simulink model "TST_InjSys_CtlQnt"  (R2016b)
settings: Solver=FixedStepDiscrete  StartTime=0.0  StopTime=simTime  FixedStep=sampleTime  RelTol=1e-3
values from neighbouring files (symbols this model uses):
  testCase = 1    [initTST_InjSys_CtlQnt_001.m]
libraries: simulink x4, UnitTest_Lib x2
settings Model: Creator=zhengjinyan  LastModifiedBy=zhengjinyan
settings DebuggingCC: SignalRangeChecking=error

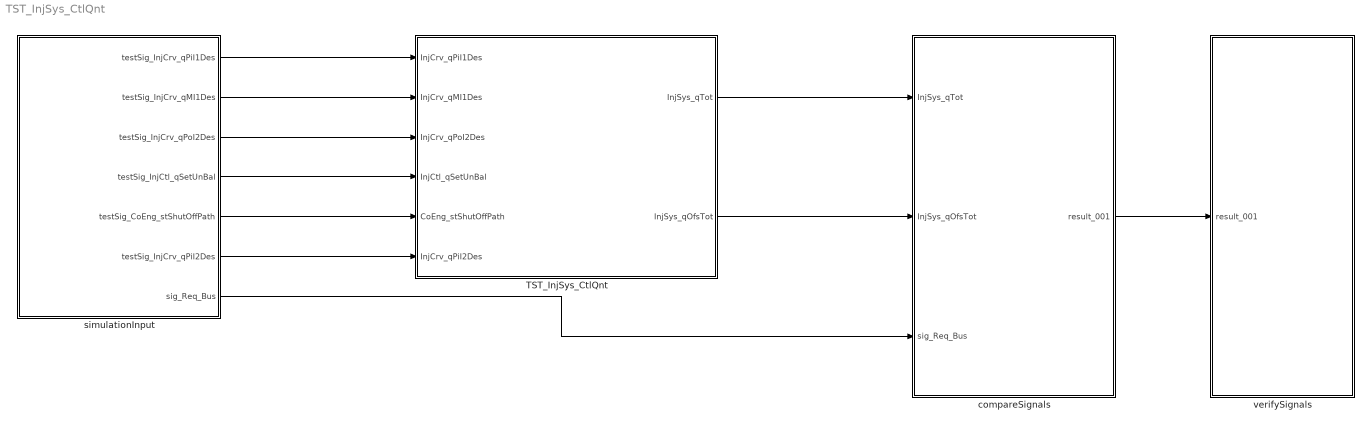
== system TST_InjSys_CtlQnt ==
  TST_InjSys_CtlQnt : Subsystem
  compareSignals : Subsystem
  simulationInput : Subsystem
  verifySignals : Subsystem
  wires:
  simulationInput/1(testSig_InjCrv_qPiI1Des) -> TST_InjSys_CtlQnt/1(InjCrv_qPiI1Des)
  simulationInput/2(testSig_InjCrv_qMI1Des) -> TST_InjSys_CtlQnt/2(InjCrv_qMI1Des)
  simulationInput/3(testSig_InjCrv_qPoI2Des) -> TST_InjSys_CtlQnt/3(InjCrv_qPoI2Des)
  simulationInput/4(testSig_InjCtl_qSetUnBal) -> TST_InjSys_CtlQnt/4(InjCtl_qSetUnBal)
  simulationInput/5(testSig_CoEng_stShutOffPath) -> TST_InjSys_CtlQnt/5(CoEng_stShutOffPath)
  simulationInput/6(testSig_InjCrv_qPiI2Des) -> TST_InjSys_CtlQnt/6(InjCrv_qPiI2Des)
  TST_InjSys_CtlQnt/1(InjSys_qTot) -> compareSignals/1(InjSys_qTot)
  TST_InjSys_CtlQnt/2(InjSys_qOfsTot) -> compareSignals/2(InjSys_qOfsTot)
  simulationInput/7(sig_Req_Bus) -> compareSignals/3(sig_Req_Bus)
  compareSignals/1(result_001) -> verifySignals/1(result_001)

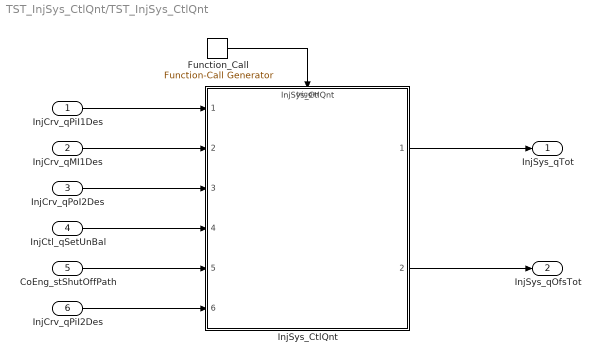
== system TST_InjSys_CtlQnt/TST_InjSys_CtlQnt ==
  InjCrv_qPiI1Des : Inport
  InjCrv_qMI1Des : Inport  Port=2
  InjCrv_qPoI2Des : Inport  Port=3
  InjCtl_qSetUnBal : Inport  Port=4
  CoEng_stShutOffPath : Inport  Port=5
  InjCrv_qPiI2Des : Inport  Port=6
  Function_Call : simulink/Ports & Subsystems/Function-Call Generator  sample_time=sampleTime  numberOfIterations=1
  InjSys_CtlQnt : ModelReference  ModelNameDialog=InjSys_CtlQnt  SimulationMode=Normal  ModelReferenceVersion=1.5  TriggerPortName=function  TriggerPortTriggerType=function-call  TriggerPortStatesWhenEnabling=held
  InjSys_qTot : Outport
  InjSys_qOfsTot : Outport  Port=2
  wires:
  Function_Call/1 -> InjSys_CtlQnt/Trigger
  InjCrv_qPiI1Des/1 -> InjSys_CtlQnt/1
  InjCrv_qMI1Des/1 -> InjSys_CtlQnt/2
  InjCrv_qPoI2Des/1 -> InjSys_CtlQnt/3
  InjCtl_qSetUnBal/1 -> InjSys_CtlQnt/4
  CoEng_stShutOffPath/1 -> InjSys_CtlQnt/5
  InjCrv_qPiI2Des/1 -> InjSys_CtlQnt/6
  InjSys_CtlQnt/1 -> InjSys_qTot/1
  InjSys_CtlQnt/2 -> InjSys_qOfsTot/1

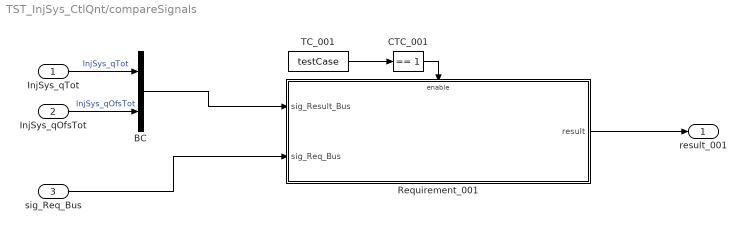
== system TST_InjSys_CtlQnt/compareSignals ==
  InjSys_qTot : Inport
  InjSys_qOfsTot : Inport  Port=2
  sig_Req_Bus : Inport  Port=3
  BC : BusCreator  Inputs=2
  CTC_001 : simulink/Logic and Bit Operations/Compare To Constant  relop===  const=1  OutDataTypeStr=boolean
  Requirement_001 : Subsystem
  TC_001 : Constant  Value=testCase
  result_001 : Outport
  wires:
  InjSys_qTot/1 -> BC/1  "InjSys_qTot"
  InjSys_qOfsTot/1 -> BC/2  "InjSys_qOfsTot"
  TC_001/1 -> CTC_001/1
  CTC_001/1 -> Requirement_001/Enable
  sig_Req_Bus/1 -> Requirement_001/2(sig_Req_Bus)
  BC/1 -> Requirement_001/1(sig_Result_Bus)
  Requirement_001/1(result) -> result_001/1

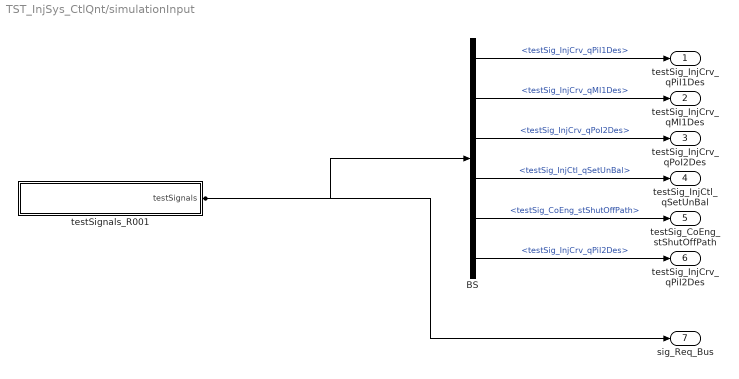
== system TST_InjSys_CtlQnt/simulationInput ==
  BS : BusSelector  OutputSignals=testSig_InjCrv_qPiI1Des,testSig_InjCrv_qMI1Des,testSig_InjCrv_qPoI2Des,testSig_InjCtl_qSetUnBal,testSig_CoEng_stShutOffPath,testSig_InjCrv_qPiI2Des
  testSignals_R001 : Subsystem
  testSig_InjCrv_qPiI1Des : Outport
  testSig_InjCrv_qMI1Des : Outport  Port=2
  testSig_InjCrv_qPoI2Des : Outport  Port=3
  testSig_InjCtl_qSetUnBal : Outport  Port=4
  testSig_CoEng_stShutOffPath : Outport  Port=5
  testSig_InjCrv_qPiI2Des : Outport  Port=6
  sig_Req_Bus : Outport  Port=7
  wires:
  BS/1 -> testSig_InjCrv_qPiI1Des/1  "<testSig_InjCrv_qPiI1Des>"
  BS/2 -> testSig_InjCrv_qMI1Des/1  "<testSig_InjCrv_qMI1Des>"
  BS/3 -> testSig_InjCrv_qPoI2Des/1  "<testSig_InjCrv_qPoI2Des>"
  BS/4 -> testSig_InjCtl_qSetUnBal/1  "<testSig_InjCtl_qSetUnBal>"
  BS/5 -> testSig_CoEng_stShutOffPath/1  "<testSig_CoEng_stShutOffPath>"
  BS/6 -> testSig_InjCrv_qPiI2Des/1  "<testSig_InjCrv_qPiI2Des>"
  testSignals_R001/1(testSignals) -> BS/1, sig_Req_Bus/1

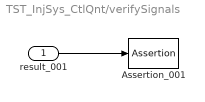
== system TST_InjSys_CtlQnt/verifySignals ==
  result_001 : Inport
  Assertion_001 : Assertion  Enabled=off
  wires:
  result_001/1 -> Assertion_001/1

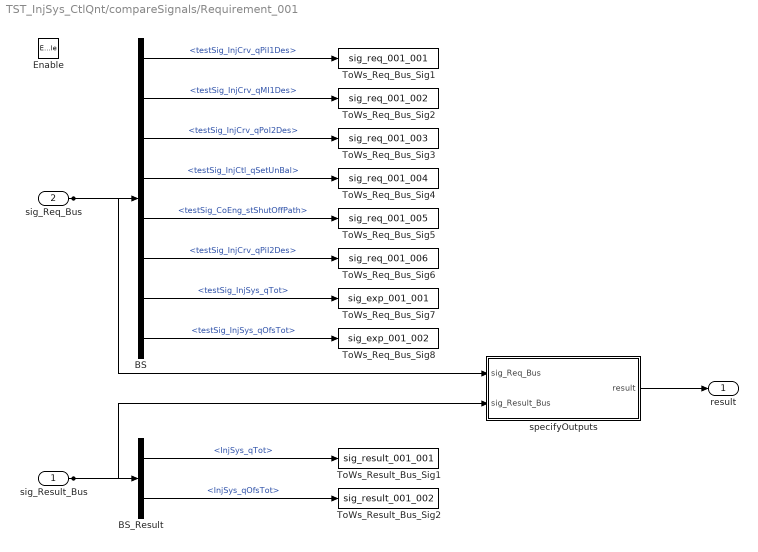
== system TST_InjSys_CtlQnt/compareSignals/Requirement_001 ==
  sig_Result_Bus : Inport
  sig_Req_Bus : Inport  Port=2
  Enable : EnablePort
  BS : BusSelector  OutputSignals=testSig_InjCrv_qPiI1Des,testSig_InjCrv_qMI1Des,testSig_InjCrv_qPoI2Des,testSig_InjCtl_qSetUnBal,testSig_CoEng_stShutOffPath,testSig_InjCrv_qPiI2Des,testSig_InjSys_qTot,testSig_InjSys_qOfsTot
  BS_Result : BusSelector  OutputSignals=InjSys_qTot,InjSys_qOfsTot
  ToWs_Req_Bus_Sig1 : ToWorkspace  VariableName=sig_req_001_001  SaveFormat=Structure With Time
  ToWs_Req_Bus_Sig2 : ToWorkspace  VariableName=sig_req_001_002  SaveFormat=Structure With Time
  ToWs_Req_Bus_Sig3 : ToWorkspace  VariableName=sig_req_001_003  SaveFormat=Structure With Time
  ToWs_Req_Bus_Sig4 : ToWorkspace  VariableName=sig_req_001_004  SaveFormat=Structure With Time
  ToWs_Req_Bus_Sig5 : ToWorkspace  VariableName=sig_req_001_005  SaveFormat=Structure With Time
  ToWs_Req_Bus_Sig6 : ToWorkspace  VariableName=sig_req_001_006  SaveFormat=Structure With Time
  ToWs_Req_Bus_Sig7 : ToWorkspace  VariableName=sig_exp_001_001  SaveFormat=Structure With Time
  ToWs_Req_Bus_Sig8 : ToWorkspace  VariableName=sig_exp_001_002  SaveFormat=Structure With Time
  ToWs_Result_Bus_Sig1 : ToWorkspace  VariableName=sig_result_001_001  SaveFormat=Structure With Time
  ToWs_Result_Bus_Sig2 : ToWorkspace  VariableName=sig_result_001_002  SaveFormat=Structure With Time
  specifyOutputs : Subsystem
  result : Outport
  wires:
  sig_Req_Bus/1 -> BS/1, specifyOutputs/1(sig_Req_Bus)
  BS/1 -> ToWs_Req_Bus_Sig1/1  "<testSig_InjCrv_qPiI1Des>"
  BS/2 -> ToWs_Req_Bus_Sig2/1  "<testSig_InjCrv_qMI1Des>"
  BS/3 -> ToWs_Req_Bus_Sig3/1  "<testSig_InjCrv_qPoI2Des>"
  BS/4 -> ToWs_Req_Bus_Sig4/1  "<testSig_InjCtl_qSetUnBal>"
  BS/5 -> ToWs_Req_Bus_Sig5/1  "<testSig_CoEng_stShutOffPath>"
  BS/6 -> ToWs_Req_Bus_Sig6/1  "<testSig_InjCrv_qPiI2Des>"
  BS/7 -> ToWs_Req_Bus_Sig7/1  "<testSig_InjSys_qTot>"
  BS/8 -> ToWs_Req_Bus_Sig8/1  "<testSig_InjSys_qOfsTot>"
  sig_Result_Bus/1 -> BS_Result/1, specifyOutputs/2(sig_Result_Bus)
  BS_Result/1 -> ToWs_Result_Bus_Sig1/1  "<InjSys_qTot>"
  BS_Result/2 -> ToWs_Result_Bus_Sig2/1  "<InjSys_qOfsTot>"
  specifyOutputs/1(result) -> result/1

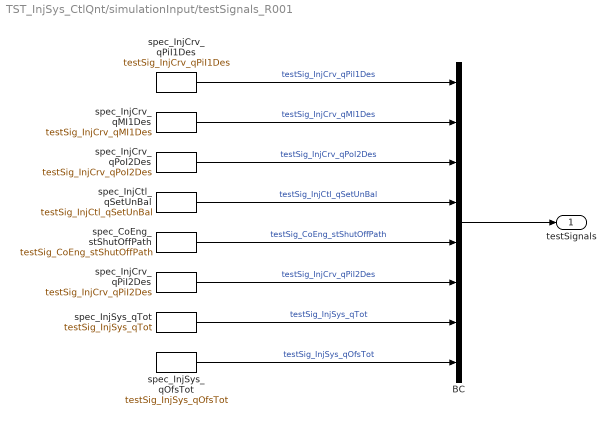
== system TST_InjSys_CtlQnt/simulationInput/testSignals_R001 ==
  BC : BusCreator  Inputs=8
  spec_CoEng_stShutOffPath : FromWorkspace  VariableName=testSig_CoEng_stShutOffPath  Interpolate=off  OutputAfterFinalValue=Holding final value
  spec_InjCrv_qMI1Des : FromWorkspace  VariableName=testSig_InjCrv_qMI1Des  Interpolate=off  OutputAfterFinalValue=Holding final value
  spec_InjCrv_qPiI1Des : FromWorkspace  VariableName=testSig_InjCrv_qPiI1Des  Interpolate=off  OutputAfterFinalValue=Holding final value
  spec_InjCrv_qPiI2Des : FromWorkspace  VariableName=testSig_InjCrv_qPiI2Des  Interpolate=off  OutputAfterFinalValue=Holding final value
  spec_InjCrv_qPoI2Des : FromWorkspace  VariableName=testSig_InjCrv_qPoI2Des  Interpolate=off  OutputAfterFinalValue=Holding final value
  spec_InjCtl_qSetUnBal : FromWorkspace  VariableName=testSig_InjCtl_qSetUnBal  Interpolate=off  OutputAfterFinalValue=Holding final value
  spec_InjSys_qOfsTot : FromWorkspace  VariableName=testSig_InjSys_qOfsTot  Interpolate=off  OutputAfterFinalValue=Holding final value
  spec_InjSys_qTot : FromWorkspace  VariableName=testSig_InjSys_qTot  Interpolate=off  OutputAfterFinalValue=Holding final value
  testSignals : Outport
  wires:
  BC/1 -> testSignals/1
  spec_InjCrv_qPiI1Des/1 -> BC/1  "testSig_InjCrv_qPiI1Des"
  spec_InjCrv_qMI1Des/1 -> BC/2  "testSig_InjCrv_qMI1Des"
  spec_InjCrv_qPoI2Des/1 -> BC/3  "testSig_InjCrv_qPoI2Des"
  spec_InjCtl_qSetUnBal/1 -> BC/4  "testSig_InjCtl_qSetUnBal"
  spec_CoEng_stShutOffPath/1 -> BC/5  "testSig_CoEng_stShutOffPath"
  spec_InjCrv_qPiI2Des/1 -> BC/6  "testSig_InjCrv_qPiI2Des"
  spec_InjSys_qTot/1 -> BC/7  "testSig_InjSys_qTot"
  spec_InjSys_qOfsTot/1 -> BC/8  "testSig_InjSys_qOfsTot"

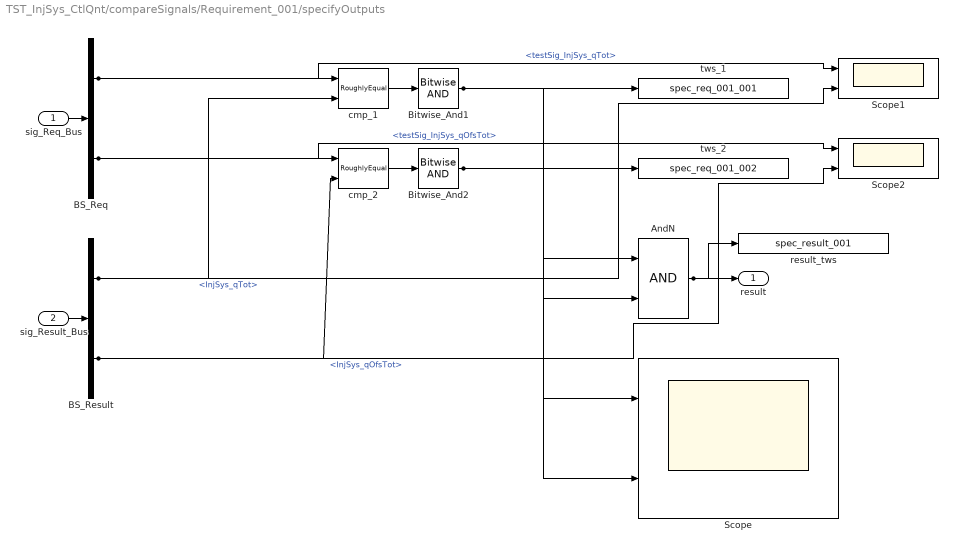
== system TST_InjSys_CtlQnt/compareSignals/Requirement_001/specifyOutputs ==
  sig_Req_Bus : Inport
  sig_Result_Bus : Inport  Port=2
  AndN : Logic
  BS_Req : BusSelector  OutputSignals=testSig_InjSys_qTot,testSig_InjSys_qOfsTot
  BS_Result : BusSelector  OutputSignals=InjSys_qTot,InjSys_qOfsTot
  Bitwise_And1 : simulink/Logic and Bit Operations/Bitwise Operator  logicop=AND  UseBitMask=off  BitMask=bin2dec('11011001')  BitMaskRealWorld=Stored Integer
  Bitwise_And2 : simulink/Logic and Bit Operations/Bitwise Operator  logicop=AND  UseBitMask=off  BitMask=bin2dec('11011001')  BitMaskRealWorld=Stored Integer
  Scope : Scope  NumInputPorts=2
  Scope1 : Scope  NumInputPorts=2
  Scope2 : Scope  NumInputPorts=2
  cmp_1 : UnitTest_Lib/RoughlyEqual  slope=0.1
  cmp_2 : UnitTest_Lib/RoughlyEqual  slope=0.1
  result_tws : ToWorkspace  VariableName=spec_result_001
  tws_1 : ToWorkspace  VariableName=spec_req_001_001
  tws_2 : ToWorkspace  VariableName=spec_req_001_002
  result : Outport
  wires:
  sig_Req_Bus/1 -> BS_Req/1
  sig_Result_Bus/1 -> BS_Result/1
  AndN/1 -> result/1, result_tws/1
  BS_Req/1 -> cmp_1/1, Scope1/1  "<testSig_InjSys_qTot>"
  BS_Result/1 -> cmp_1/2, Scope1/2  "<InjSys_qTot>"
  cmp_1/1 -> Bitwise_And1/1
  Bitwise_And1/1 -> tws_1/1, AndN/1, Scope/1
  BS_Req/2 -> cmp_2/1, Scope2/1  "<testSig_InjSys_qOfsTot>"
  BS_Result/2 -> cmp_2/2, Scope2/2  "<InjSys_qOfsTot>"
  cmp_2/1 -> Bitwise_And2/1
  Bitwise_And2/1 -> tws_2/1, AndN/2, Scope/2
